simulink model "moonrir"  (R2024b)
settings: Solver=VariableStepAuto  StartTime=0.0  StopTime=10.0  RelTol=1e-3
libraries: arduinolib x4, simulink x1

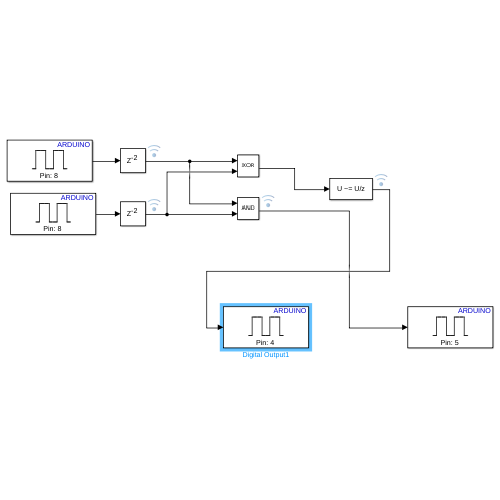
[thumbnail: Simulink's stored preview of the top-level diagram]
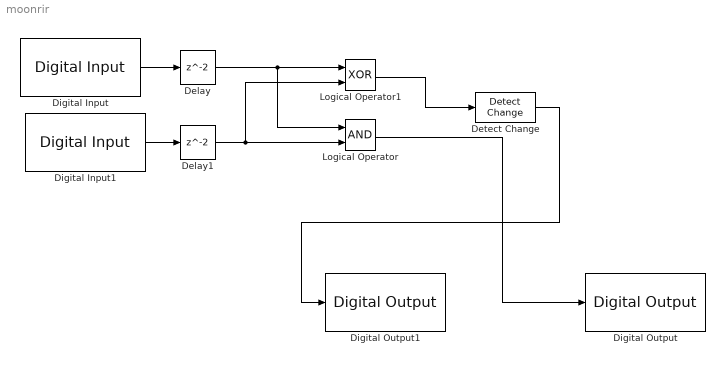
== system moonrir ==
  Delay : Delay
  Delay1 : Delay
  Detect Change : simulink/Logic and Bit Operations/Detect Change  vinit=0  OutDataTypeStr=boolean
  Digital Input : arduinolib/Digital Input  pinNumber=8  mode=Default  Direction=input  SampleTime=0.1  blockPlatform=arduino
      settings: SourceProductName=Common
  Digital Input1 : arduinolib/Digital Input  pinNumber=8  mode=Default  Direction=input  SampleTime=0.1  blockPlatform=arduino
      settings: SourceProductName=Common
  Digital Output : arduinolib/Digital Output  pinNumber=5  Direction=output  blockPlatform=arduino
      settings: SourceProductName=Common
  Digital Output1 : arduinolib/Digital Output  pinNumber=4  Direction=output  blockPlatform=arduino
      settings: SourceProductName=Common
  Logical Operator : Logic  AllPortsSameDT=off  OutDataTypeStr=boolean
  Logical Operator1 : Logic  Operator=XOR  AllPortsSameDT=off  OutDataTypeStr=boolean
  wires:
  Digital Input/1 -> Delay/1
  Digital Input1/1 -> Delay1/1
  Delay/1 -> Logical Operator/1, Logical Operator1/1
  Delay1/1 -> Logical Operator1/2, Logical Operator/2
  Logical Operator1/1 -> Detect Change/1
  Detect Change/1 -> Digital Output1/1
  Logical Operator/1 -> Digital Output/1
